simulink model "sw_rate_limiter"  (R2016b)
settings: Solver=VariableStepAuto  StartTime=0.0  StopTime=10.0  RelTol=1e-3
undefined symbols (not defined in the file or in its folder): A_butter, B_butter, C_butter, D_butter
settings Model: Creator=nicol  LastModifiedBy=nicol

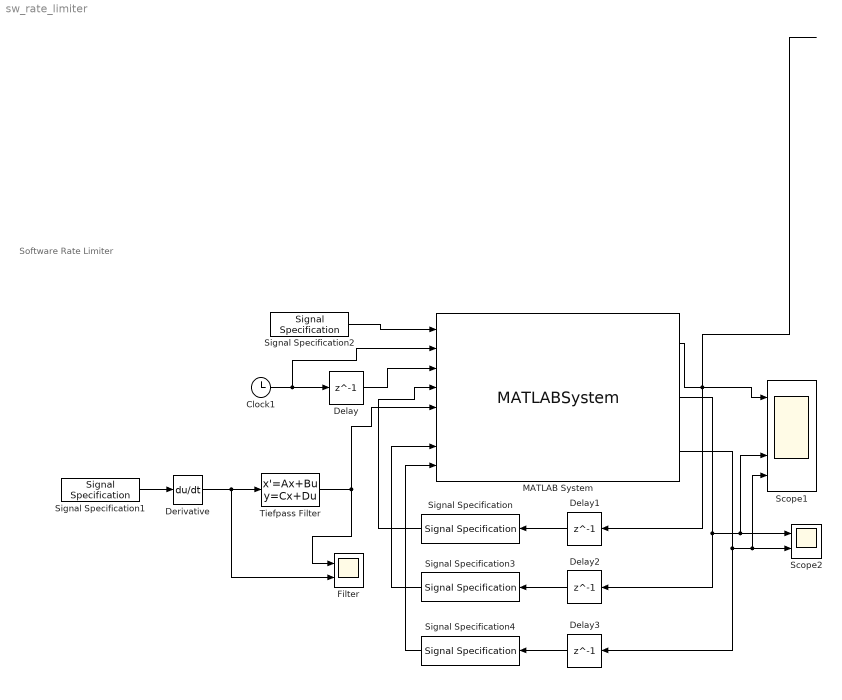
== system sw_rate_limiter ==
  note: Software Rate Limiter
  Clock1 : Clock
  Delay{,1..3} (4 alike) : Delay  DelayLength=1
  Derivative : Derivative
  Filter : Scope  NumInputPorts=2
  MATLAB System : MATLABSystem  System=rate_limiter_classdef  SimulateUsing=Code generation
      mask Type: rate_limiter_classdef
      mask Display:
      | disp('rate_limiter_classdef');
      | port_label('input',1,'input');
      | port_label('input',2,'clock');
      | port_label('input',3,'clock_delayed');
      | port_label('input',4,'last_value');
      | port_label('input',5,'deriv');
      | port_label('input',6,'rate_limiter');
      | port_label('input',7,'rl_integral_in');
      | port_label('input',8,'rl_groesser_y_in');
      | port_label('output',1,'y');
      | port_label('output',2,'rl_integral_out');
      | port_label('output',3,'rl_groesser_y_out');
  Scope1 : Scope  NumInputPorts=5
  Scope2 : Scope  NumInputPorts=2
  Signal Specification : SignalSpecification  OutDataTypeStr=double  Dimensions=1
  Signal Specification1 : SignalSpecification  Dimensions=1
  Signal Specification2 : SignalSpecification  Dimensions=1
  Signal Specification3 : SignalSpecification  OutDataTypeStr=double  Dimensions=1
  Signal Specification4 : SignalSpecification  OutDataTypeStr=double  Dimensions=1
  Tiefpass Filter : StateSpace  A=A_butter  B=B_butter  C=C_butter  D=D_butter  X0=0
  wires:
  ? -> Signal Specification1/1, Signal Specification2/1, Scope1/3
  Clock1/1 -> MATLAB System/2, Delay/1
  Delay/1 -> MATLAB System/3
  Delay1/1 -> Signal Specification/1
  Signal Specification/1 -> MATLAB System/4
  Signal Specification2/1 -> MATLAB System/1
  Signal Specification1/1 -> Derivative/1
  Derivative/1 -> Filter/2, Tiefpass Filter/1
  Tiefpass Filter/1 -> Filter/1, MATLAB System/5
  MATLAB System/1 -> Delay1/1, Scope1/1
  Delay2/1 -> Signal Specification3/1
  Delay3/1 -> Signal Specification4/1
  MATLAB System/2 -> Scope1/4, Scope2/1, Delay2/1
  MATLAB System/3 -> Scope1/5, Scope2/2, Delay3/1
  Signal Specification3/1 -> MATLAB System/7
  Signal Specification4/1 -> MATLAB System/8
  ? -> MATLAB System/6
  ? -> Scope1/2
